simulink model "SatelliteServicing_3LinkPlanar - Copy"  (R2021a)
settings: Solver=ode15s  StartTime=0.0  StopTime=endTime  RelTol=1e-3
undefined symbols (not defined in the file or in its folder): alpha, Base_a, Base_c, Base_z, client, controlData, DiscIntNeverNeededParam, inertiaMat, inertiaMatBase, Link_Length, linkInertia, massVec, mt, nav, rod, sat, sigbuilder_block, smiData, X, Y, Z
libraries: nesl_utility x113, sm_lib x56
(part 3 of 3)

== system SatelliteServicing_3LinkPlanar - Copy/ServicingSatellite/SatSolarPanel2 ==
  Rigid Transform : sm_lib/Frames and Transforms/Rigid Transform  TranslationMethod=None  TranslationStandardOffset=0  TranslationLengthUnit=m  TranslationStandardAxis=+Z  TranslationCartesianOffset=[0 0 0]  TranslationROffset=0  TranslationROffsetUnits=m  TranslationZOffset=0  TranslationZOffsetUnits=m  TranslationThetaOffset=0  TranslationThetaOffsetUnits=deg  RotationMethod=RotationSequence  RotationAngleUnits=deg  RotationStandardAxis=+Z  RotationAngle=0.0  RotationArbitraryAxis=[0 0 1]  FollAlignAxisA=+X  BaseAlignAxisA=+Y  FollAlignAxisB=+Y  BaseAlignAxisB=+Z  RotationSequenceAxes=FollowerAxes  RotationSequence=YZX  RotationSequenceAngles=[0 90 0]  RotationSequenceAnglesUnits=deg  RotationMatrix=[1 0 0; 0 1 0; 0 0 1]
  SolarPanelSolid1 : sm_lib/Body Elements/Brick Solid  GraphicAmbientColor=[0.15 0.15 0.15 1.0]  BasedOnType=Mass  BrickDimensions=sat.service.panel_mount.dim  BrickDimensionUnits=m  CenterOfMass=[0 0 0]  CenterOfMassUnits=m  GraphicDiffuseColor=[0.2 0.2 0.2]  Density=1000  DensityUnits=kg/m^3  DoExposeReferenceFrame=off  GraphicEmissiveColor=[0.0 0.0 0.0 1.0]  ExportEntireGeometry=off  SerializedFrames=<Frames><Frame><Id>Frame1</Id><Value><Name>F1</Name><Origin><Source>GeometricFeature</Source><FeatureName>-x surface</FeatureName></Origin><PrimaryAxis><DefinedDirection>+Z</DefinedDirection><Source>ReferenceFrame</Source><SourceDirection>+Z</SourceDirection><FeatureName></FeatureName></PrimaryAxis><SecondaryAxis><DefinedDirection>+X</DefinedDirection><Source>ReferenceFrame</Source><SourceDirection>+X</SourceDirection><FeatureName></FeatureName></SecondaryAxis></Value></Frame><Frame><Id>Frame2</Id><Value><Name>F2</Name><Origin><Source>GeometricFeature</Source><FeatureName>+x surface</FeatureName></Origin><PrimaryAxis><DefinedDirection>+Z</DefinedDirection><Source>ReferenceFrame</Source><SourceDirection>+Z</SourceDirection><FeatureName></FeatureName></PrimaryAxis><SecondaryAxis><DefinedDirection>+X</DefinedDirection><Source>ReferenceFrame</Source><SourceDirection>+X</SourceDirection><FeatureName></FeatureName></SecondaryAxis></Value></Frame></Frames>  MarkerShape=Sphere  MarkerSize=10  GraphicType=FromGeometry  InertiaType=CalculateFromGeometry  Mass=sat.service.panel_mount.mass  MassUnits=kg  MomentsOfInertia=[1 1 1]  MomentsOfInertiaUnits=kg*m^2  GraphicOpacity=0.5  ProductsOfInertia=[0 0 0]  ProductsOfInertiaUnits=kg*m^2  GraphicShininess=75  GraphicSpecularColor=[0.5 0.5 0.5 1.0]  GraphicVisPropType=SimpleVisualProperties
  SolarPanelSolid2 : sm_lib/Body Elements/Brick Solid  GraphicAmbientColor=[0.15 0.15 0.15 1.0]  BasedOnType=Mass  BrickDimensions=sat.service.panel.dim  BrickDimensionUnits=m  CenterOfMass=[0 0 0]  CenterOfMassUnits=m  GraphicDiffuseColor=[0.0 0.2 0.8]  Density=1000  DensityUnits=kg/m^3  DoExposeReferenceFrame=off  GraphicEmissiveColor=[0.0 0.0 0.0 1.0]  ExportEntireGeometry=off  SerializedFrames=<Frames><Frame><Id>Frame1</Id><Value><Name>F1</Name><Origin><Source>GeometricFeature</Source><FeatureName>-x surface</FeatureName></Origin><PrimaryAxis><DefinedDirection>+Z</DefinedDirection><Source>ReferenceFrame</Source><SourceDirection>+Z</SourceDirection><FeatureName></FeatureName></PrimaryAxis><SecondaryAxis><DefinedDirection>+X</DefinedDirection><Source>ReferenceFrame</Source><SourceDirection>+X</SourceDirection><FeatureName></FeatureName></SecondaryAxis></Value></Frame></Frames>  MarkerShape=Sphere  MarkerSize=10  GraphicType=FromGeometry  InertiaType=CalculateFromGeometry  Mass=sat.service.panel.mass  MassUnits=kg  MomentsOfInertia=[1 1 1]  MomentsOfInertiaUnits=kg*m^2  GraphicOpacity=0.5  ProductsOfInertia=[0 0 0]  ProductsOfInertiaUnits=kg*m^2  GraphicShininess=75  GraphicSpecularColor=[0.5 0.5 0.5 1.0]  GraphicVisPropType=SimpleVisualProperties
  F1 : PMIOPort  Side=Left
  connections:
  SolarPanelSolid2/LConn1 -- SolarPanelSolid1/RConn1
  Rigid Transform/RConn1 -- SolarPanelSolid1/LConn1
  Rigid Transform/LConn1 -- F1/RConn1

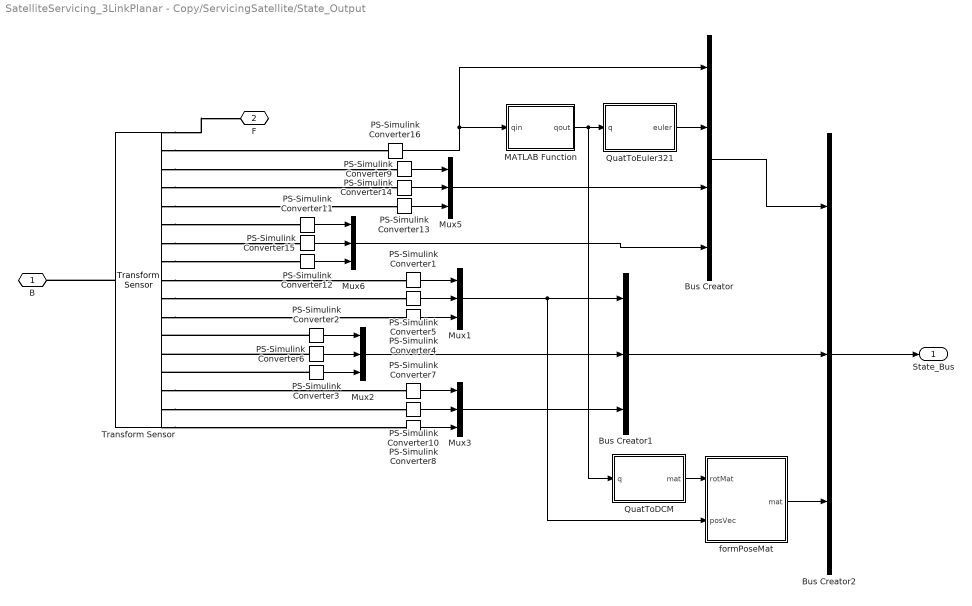
== system SatelliteServicing_3LinkPlanar - Copy/ServicingSatellite/State_Output ==
  Bus Creator : BusCreator  Inputs=4  OutDataTypeStr=Bus: RotStateBus
      settings: InheritFromInputs=off
  Bus Creator1 : BusCreator  Inputs=3  OutDataTypeStr=Bus: TransStateBus
      settings: InheritFromInputs=off
  Bus Creator2 : BusCreator  Inputs=3  OutDataTypeStr=Bus: StateBus
      settings: InheritFromInputs=off
  MATLAB Function : MATLAB Function  TreatAsAtomicUnit=on
  Mux{1..3,5..6} (5 alike) : Mux  Inputs=3
  PS-Simulink Converter{1..16} (16 alike) : nesl_utility/PS-Simulink Converter  PhysicalDomain=network_engine_domain  SubClassName=ps_output  LeftPortType=input  RightPortType=output  PseudoPeriodic=off  Frequencies=[]  Unit=inherit  AffineConversion=off
      settings: SourceProductBaseCode=PW,SS
  QuatToDCM : MATLAB Function  TreatAsAtomicUnit=on
  QuatToEuler321 : MATLAB Function  TreatAsAtomicUnit=on
  Transform Sensor : sm_lib/Frames and Transforms/Transform Sensor  MeasurementFrame=World  SenseAngle=off  SenseAxis=off  SenseAngle1=off  SenseAngle2=off  SenseAngle3=off  SenseQ=on  SenseR=off  SenseOmegaX=on  SenseOmegaY=on  SenseOmegaZ=on  SenseOmega1=off  SenseOmega2=off  SenseOmega3=off  SenseQDot=off  SenseRDot=off  SenseAlphaX=on  SenseAlphaY=on  SenseAlphaZ=on  SenseAlpha1=off  SenseAlpha2=off  SenseAlpha3=off  SenseQDDot=off  SenseRDDot=off  SenseX=on  SenseY=on  SenseZ=on  SenseRad=off  SenseAzim=off  SenseDist=off  SenseInc=off  SenseXDot=on  SenseYDot=on  SenseZDot=on  SenseRadDot=off  SenseAzimDot=off  SenseDistDot=off  SenseIncDot=off  SenseXDDot=on  SenseYDDot=on  SenseZDDot=on  SenseRadDDot=off  SenseAzimDDot=off  SenseDistDDot=off  SenseIncDDot=off
  formPoseMat : MATLAB Function  TreatAsAtomicUnit=on
  B : PMIOPort  Side=Left
  F : PMIOPort  Port=2  Side=Right
  State_Bus : Outport
  wires:
  PS-Simulink Converter4/1 -> Mux1/3
  PS-Simulink Converter5/1 -> Mux1/2
  PS-Simulink Converter1/1 -> Mux1/1
  PS-Simulink Converter3/1 -> Mux2/3
  PS-Simulink Converter6/1 -> Mux2/2
  PS-Simulink Converter2/1 -> Mux2/1
  PS-Simulink Converter10/1 -> Mux3/2
  PS-Simulink Converter8/1 -> Mux3/3
  PS-Simulink Converter7/1 -> Mux3/1
  Mux2/1 -> Bus Creator1/2
  Mux1/1 -> formPoseMat/2(posVec), Bus Creator1/1
  Mux3/1 -> Bus Creator1/3
  PS-Simulink Converter9/1 -> Mux5/1
  PS-Simulink Converter14/1 -> Mux5/2
  PS-Simulink Converter13/1 -> Mux5/3
  Mux5/1 -> Bus Creator/3
  PS-Simulink Converter15/1 -> Mux6/2
  PS-Simulink Converter12/1 -> Mux6/3
  Mux6/1 -> Bus Creator/4
  PS-Simulink Converter11/1 -> Mux6/1
  PS-Simulink Converter16/1 -> Bus Creator/1, MATLAB Function/1(qin)
  QuatToEuler321/1(euler) -> Bus Creator/2
  Bus Creator/1 -> Bus Creator2/1
  Bus Creator1/1 -> Bus Creator2/2
  Bus Creator2/1 -> State_Bus/1
  MATLAB Function/1(qout) -> QuatToDCM/1(q), QuatToEuler321/1(q)
  QuatToDCM/1(mat) -> formPoseMat/1(rotMat)
  formPoseMat/1(mat) -> Bus Creator2/3
  connections:
  Transform Sensor/LConn1 -- B/RConn1
  Transform Sensor/RConn1 -- F/RConn1
  Transform Sensor/RConn9 -- PS-Simulink Converter1/LConn1
  Transform Sensor/RConn10 -- PS-Simulink Converter5/LConn1
  Transform Sensor/RConn11 -- PS-Simulink Converter4/LConn1
  PS-Simulink Converter3/LConn1 -- Transform Sensor/RConn14
  PS-Simulink Converter6/LConn1 -- Transform Sensor/RConn13
  PS-Simulink Converter2/LConn1 -- Transform Sensor/RConn12
  Transform Sensor/RConn17 -- PS-Simulink Converter8/LConn1
  Transform Sensor/RConn15 -- PS-Simulink Converter7/LConn1
  Transform Sensor/RConn16 -- PS-Simulink Converter10/LConn1
  Transform Sensor/RConn8 -- PS-Simulink Converter12/LConn1
  Transform Sensor/RConn5 -- PS-Simulink Converter13/LConn1
  Transform Sensor/RConn4 -- PS-Simulink Converter14/LConn1
  Transform Sensor/RConn3 -- PS-Simulink Converter9/LConn1
  Transform Sensor/RConn7 -- PS-Simulink Converter15/LConn1
  Transform Sensor/RConn6 -- PS-Simulink Converter11/LConn1
  Transform Sensor/RConn2 -- PS-Simulink Converter16/LConn1

== system SatelliteServicing_3LinkPlanar - Copy/GNC/Control/MassProperties ==
  linkInertia : Inport
  Bus Creator : BusCreator  Inputs=5  OutDataTypeStr=Bus: MassPropertiesBus
      settings: InheritFromInputs=off
  Constant10 : Constant  Value=massVec
  Constant11 : Constant  Value=mt
  Constant12 : Constant  Value=inertiaMatBase
  Constant13 : Constant  Value=inertiaMat
  InitialMP : Outport
  wires:
  Constant11/1 -> Bus Creator/1
  Constant10/1 -> Bus Creator/2
  Constant12/1 -> Bus Creator/3
  Constant13/1 -> Bus Creator/4
  Bus Creator/1 -> InitialMP/1
  ? -> Bus Creator/5

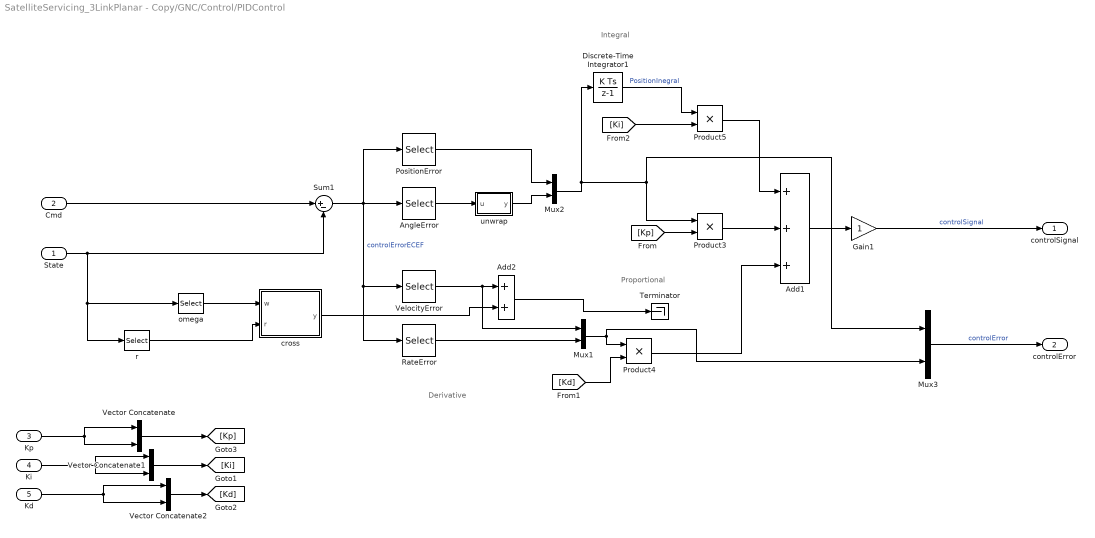
== system SatelliteServicing_3LinkPlanar - Copy/GNC/Control/PIDControl ==
  note: Derivative
  note: Proportional
  note: Integral
  State : Inport
  Cmd : Inport  Port=2
  Kp : Inport  Port=3
  Ki : Inport  Port=4
  Kd : Inport  Port=5
  Add1 : Sum  Inputs=+++
  Add2 : Sum
  AngleError : Selector  IndexOptions=Index vector (dialog)  Indices=[4:6]  OutputSizes=1
  Discrete-Time Integrator1 : DiscreteIntegrator  SampleTime=-1  ICPrevOutput=DiscIntNeverNeededParam  ICPrevScaledInput=DiscIntNeverNeededParam
  Gain1 : Gain
  Mux1 : Mux  Inputs=2
  Mux2 : Mux  Inputs=2
  Mux3 : Mux  Inputs=2
  PositionError : Selector  IndexOptions=Index vector (dialog)  Indices=[1:3]  OutputSizes=1
  Product3 : Product
  Product4 : Product
  Product5 : Product
  RateError : Selector  IndexOptions=Index vector (dialog)  Indices=[10:12]  OutputSizes=1
  Sum1 : Sum  Inputs=|+-
  Terminator : Terminator
  Vector Concatenate : Concatenate
  Vector Concatenate1 : Concatenate
  Vector Concatenate2 : Concatenate
  VelocityError : Selector  IndexOptions=Index vector (dialog)  Indices=[7:9]  OutputSizes=1
  cross : MATLAB Function  TreatAsAtomicUnit=on
  omega : Selector  IndexOptions=Index vector (dialog)  Indices=[10:12]  OutputSizes=1
  r : Selector  IndexOptions=Index vector (dialog)  Indices=[1:3]  OutputSizes=1
  unwrap : MATLAB Function  TreatAsAtomicUnit=on
  controlSignal : Outport
  controlError : Outport  Port=2
  wires:
  Mux2/1 -> Discrete-Time Integrator1/1, Product3/1, Mux3/1
  Product3/1 -> Add1/2
  Sum1/1 -> VelocityError/1, RateError/1, AngleError/1, PositionError/1  "controlErrorECEF"
  Discrete-Time Integrator1/1 -> Product5/1  "PositionInegral"
  RateError/1 -> Mux1/2
  Product5/1 -> Add1/1
  State/1 -> r/1, omega/1, Sum1/2
  Gain1/1 -> controlSignal/1  "controlSignal"
  cross/1(y) -> Add2/2
  PositionError/1 -> Mux2/1
  Mux1/1 -> Product4/1, Mux3/2
  Mux3/1 -> controlError/1  "controlError"
  [Ki] -> Product5/2
  r/1 -> cross/2(r)
  [Kp] -> Product3/2
  [Kd] -> Product4/2
  AngleError/1 -> unwrap/1(u)
  omega/1 -> cross/1(w)
  Add1/1 -> Gain1/1
  Product4/1 -> Add1/3
  Cmd/1 -> Sum1/1
  VelocityError/1 -> Mux1/1, Add2/1
  Kp/1 -> Vector Concatenate/1, Vector Concatenate/2
  Vector Concatenate/1 -> [Kp]
  Vector Concatenate2/1 -> [Kd]
  Kd/1 -> Vector Concatenate2/2, Vector Concatenate2/1
  Vector Concatenate1/1 -> [Ki]
  Ki/1 -> Vector Concatenate1/2, Vector Concatenate1/1
  Add2/1 -> Terminator/1
  unwrap/1(y) -> Mux2/2

== system SatelliteServicing_3LinkPlanar - Copy/GNC/Motion Inputs/SatMotion_fz ==
  Demux : Demux  Tag=STV Demux  Outputs=1
      settings: DisplayOption=none
  FromWs : FromWorkspace  Tag=STV FromWs  VariableName=tuvar
      SigBuilderData=|
      | common.afterFinalStr = 'Extrapolate'
      | common.sampleTime = 0
      | dataSet.timeRange = [0 13]
      | dataSet.name = 'Group 1'
      | sbobj.Groups.Name = 'Group 1'
      | sbobj.Groups.Signals.Name = 'SatMotion_fz'
      | sbobj.Groups.Signals.XData = [0 1 1 1.5 1.5 13]
      | sbobj.Groups.Signals.YData = [0 0 20 20 0 0]
      | sbobj.Groups.TimeRange = [0 13]
  SatMotion_fz : Outport  Tag=STV Outport
  wires:
  FromWs/1 -> Demux/1
  Demux/1 -> SatMotion_fz/1

== system SatelliteServicing_3LinkPlanar - Copy/GNC/Navigation/ComputeRelativePose ==
  Rel_to_Camera : Inport
  Bus Selector2 : BusSelector  OutputSignals=poseMatrix
  Constant1 : Constant  Value=nav.CameraToBase.orientation
  Constant2 : Constant  Value=[0 0 0]
  Product : Product  Multiplication=Matrix(*)
  Reshape : Reshape  OutputDimensionality=Column vector (2-D)
  Selector : Selector  NumberOfDimensions=2  InputPortWidth=3  IndexOptions=Index vector (dialog),Index vector (dialog)  Indices=[1:3],[1:3]  OutputSizes=1,1
  To Workspace1 : ToWorkspace  VariableName=euler_cameraAttach  SaveFormat=Timeseries  SampleTime=-1
  To Workspace2 : ToWorkspace  VariableName=mat_cameraBody  SaveFormat=Timeseries  SampleTime=-1
  formPoseMat : MATLAB Function  TreatAsAtomicUnit=on
  formRotMat : MATLAB Function  TreatAsAtomicUnit=on
  formRotMat1 : MATLAB Function  TreatAsAtomicUnit=on
  "Rel_to_CameraAttach " : Outport
  wires:
  formRotMat/1(mat) -> To Workspace2/1, formPoseMat/1(rotMat)
  Rel_to_Camera/1 -> Bus Selector2/1
  Product/1 -> Selector/1, "Rel_to_CameraAttach "/1
  Selector/1 -> formRotMat1/1(mat)
  formRotMat1/1(euler) -> To Workspace1/1
  Constant2/1 -> Reshape/1
  Reshape/1 -> formPoseMat/2(posVec)
  Constant1/1 -> formRotMat/1(euler)
  formPoseMat/1(mat) -> Product/2
  Bus Selector2/1 -> Product/1  "<poseMatrix>"

== system SatelliteServicing_3LinkPlanar - Copy/RoboticArm/ArmSegmentAssembly_2/ArmSegment_1_RIGID ==
  ReferenceFrame : sm_lib/Frames and Transforms/Reference Frame
  Solid : sm_lib/Body Elements/File Solid  ExtGeomFileName=ArmSegment_Default_sldprt.STEP  UnitType=FromFile  ExtGeomFileUnits=m  StepReaderType=HEX  ExportConvexHullGeometry=off  InertiaType=Custom  Mass=smiData.Solid(2).mass  MassUnits=kg  CenterOfMass=smiData.Solid(2).CoM  CenterOfMassUnits=mm  MomentsOfInertia=smiData.Solid(2).MoI  MomentsOfInertiaUnits=kg*mm^2  ProductsOfInertia=smiData.Solid(2).PoI  ProductsOfInertiaUnits=kg*mm^2  BasedOnType=DensityFromFile  Density=1000  DensityUnits=kg/m^3  DoExposeReferenceFrame=off  SerializedFrames=<Frames><Frame><Id>Frame1</Id><Value><Name>J1</Name><Origin><Source>GeometricFeature</Source><FeatureName>segment 68</FeatureName></Origin><PrimaryAxis><DefinedDirection>+Z</DefinedDirection><Source>ReferenceFrame</Source><SourceDirection>+Y</SourceDirection><FeatureName></FeatureName></PrimaryAxis><SecondaryAxis><DefinedDirection>+X</DefinedDirection><Source>ReferenceFrame</Source><SourceDirection>+X</SourceDirection><FeatureName></FeatureName></SecondaryAxis></Value></Frame><Frame><Id>Frame2</Id><Value><Name>J2</Name><Origin><Source>GeometricFeature</Source><FeatureName>circular curve 16</FeatureName></Origin><PrimaryAxis><DefinedDirection>+Z</DefinedDirection><Source>ReferenceFrame</Source><SourceDirection>+Y</SourceDirection><FeatureName></FeatureName></PrimaryAxis><SecondaryAxis><DefinedDirection>+X</DefinedDirection><Source>ReferenceFrame</Source><SourceDirection>+X</SourceDirection><FeatureName></FeatureName></SecondaryAxis></Value></Frame></Frames>  GraphicType=FromGeometry  MarkerShape=Sphere  MarkerSize=10  GraphicVisPropType=SimpleVisualProperties  GraphicDiffuseColor=smiData.Solid(2).color  GraphicSpecularColor=[0.5 0.5 0.5 1.0]  GraphicAmbientColor=[0.15 0.15 0.15 1.0]  GraphicEmissiveColor=[0.0 0.0 0.0 1.0]  GraphicShininess=75  GraphicOpacity=smiData.Solid(2).opacity
  Transform : sm_lib/Frames and Transforms/Rigid Transform  TranslationMethod=Cartesian  TranslationStandardOffset=0  TranslationLengthUnit=mm  TranslationStandardAxis=+Z  TranslationCartesianOffset=smiData.RigidTransform(5).translation  TranslationROffset=0  TranslationROffsetUnits=m  TranslationZOffset=0  TranslationZOffsetUnits=m  TranslationThetaOffset=0  TranslationThetaOffsetUnits=deg  RotationMethod=ArbitraryAxis  RotationAngleUnits=rad  RotationStandardAxis=+Z  RotationAngle=smiData.RigidTransform(5).angle  RotationArbitraryAxis=smiData.RigidTransform(5).axis  FollAlignAxisA=+X  BaseAlignAxisA=+Y  FollAlignAxisB=+Y  BaseAlignAxisB=+Z  RotationSequenceAxes=FollowerAxes  RotationSequence=XYX  RotationSequenceAngles=[0 0 0]  RotationSequenceAnglesUnits=deg  RotationMatrix=[1 0 0; 0 1 0; 0 0 1]
  Transform1 : sm_lib/Frames and Transforms/Rigid Transform  TranslationMethod=Cartesian  TranslationStandardOffset=0  TranslationLengthUnit=mm  TranslationStandardAxis=+Z  TranslationCartesianOffset=smiData.RigidTransform(4).translation  TranslationROffset=0  TranslationROffsetUnits=m  TranslationZOffset=0  TranslationZOffsetUnits=m  TranslationThetaOffset=0  TranslationThetaOffsetUnits=deg  RotationMethod=ArbitraryAxis  RotationAngleUnits=rad  RotationStandardAxis=+Z  RotationAngle=smiData.RigidTransform(4).angle  RotationArbitraryAxis=smiData.RigidTransform(4).axis  FollAlignAxisA=+X  BaseAlignAxisA=+Y  FollAlignAxisB=+Y  BaseAlignAxisB=+Z  RotationSequenceAxes=FollowerAxes  RotationSequence=XYX  RotationSequenceAngles=[0 0 0]  RotationSequenceAnglesUnits=deg  RotationMatrix=[1 0 0; 0 1 0; 0 0 1]
  J1_2 : PMIOPort  Side=Left
  J2_1 : PMIOPort  Port=2  Side=Right
  connections:
  Transform/RConn1 -- J2_1/RConn1
  Transform/LConn1 -- Solid/RConn1
  J1_2/RConn1 -- Transform1/LConn1
  Solid/LConn1 -- ReferenceFrame/RConn1 -- Transform1/RConn1

== system SatelliteServicing_3LinkPlanar - Copy/RoboticArm/ArmSegmentAssembly_3/ArmSegment_1_RIGID ==
  ReferenceFrame : sm_lib/Frames and Transforms/Reference Frame
  Solid : sm_lib/Body Elements/File Solid  ExtGeomFileName=ArmSegment_Default_sldprt.STEP  UnitType=FromFile  ExtGeomFileUnits=m  StepReaderType=HEX  ExportConvexHullGeometry=off  InertiaType=Custom  Mass=smiData.Solid(3).mass  MassUnits=kg  CenterOfMass=smiData.Solid(3).CoM  CenterOfMassUnits=mm  MomentsOfInertia=smiData.Solid(3).MoI  MomentsOfInertiaUnits=kg*mm^2  ProductsOfInertia=smiData.Solid(3).PoI  ProductsOfInertiaUnits=kg*mm^2  BasedOnType=DensityFromFile  Density=1000  DensityUnits=kg/m^3  DoExposeReferenceFrame=off  SerializedFrames=<Frames><Frame><Id>Frame1</Id><Value><Name>J2</Name><Origin><Source>GeometricFeature</Source><FeatureName>segment 68</FeatureName></Origin><PrimaryAxis><DefinedDirection>+Z</DefinedDirection><Source>ReferenceFrame</Source><SourceDirection>+Y</SourceDirection><FeatureName></FeatureName></PrimaryAxis><SecondaryAxis><DefinedDirection>+X</DefinedDirection><Source>ReferenceFrame</Source><SourceDirection>+X</SourceDirection><FeatureName></FeatureName></SecondaryAxis></Value></Frame><Frame><Id>Frame2</Id><Value><Name>J3</Name><Origin><Source>GeometricFeature</Source><FeatureName>circular curve 13</FeatureName></Origin><PrimaryAxis><DefinedDirection>+Z</DefinedDirection><Source>ReferenceFrame</Source><SourceDirection>+Y</SourceDirection><FeatureName></FeatureName></PrimaryAxis><SecondaryAxis><DefinedDirection>+X</DefinedDirection><Source>ReferenceFrame</Source><SourceDirection>+X</SourceDirection><FeatureName></FeatureName></SecondaryAxis></Value></Frame></Frames>  GraphicType=FromGeometry  MarkerShape=Sphere  MarkerSize=10  GraphicVisPropType=SimpleVisualProperties  GraphicDiffuseColor=smiData.Solid(2).color  GraphicSpecularColor=[0.5 0.5 0.5 1.0]  GraphicAmbientColor=[0.15 0.15 0.15 1.0]  GraphicEmissiveColor=[0.0 0.0 0.0 1.0]  GraphicShininess=75  GraphicOpacity=smiData.Solid(2).opacity
  Transform : sm_lib/Frames and Transforms/Rigid Transform  TranslationMethod=Cartesian  TranslationStandardOffset=0  TranslationLengthUnit=mm  TranslationStandardAxis=+Z  TranslationCartesianOffset=smiData.RigidTransform(6).translation  TranslationROffset=0  TranslationROffsetUnits=m  TranslationZOffset=0  TranslationZOffsetUnits=m  TranslationThetaOffset=0  TranslationThetaOffsetUnits=deg  RotationMethod=ArbitraryAxis  RotationAngleUnits=rad  RotationStandardAxis=+Z  RotationAngle=smiData.RigidTransform(6).angle  RotationArbitraryAxis=smiData.RigidTransform(6).axis  FollAlignAxisA=+X  BaseAlignAxisA=+Y  FollAlignAxisB=+Y  BaseAlignAxisB=+Z  RotationSequenceAxes=FollowerAxes  RotationSequence=XYX  RotationSequenceAngles=[0 0 0]  RotationSequenceAnglesUnits=deg  RotationMatrix=[1 0 0; 0 1 0; 0 0 1]
  Transform1 : sm_lib/Frames and Transforms/Rigid Transform  TranslationMethod=Cartesian  TranslationStandardOffset=0  TranslationLengthUnit=mm  TranslationStandardAxis=+Z  TranslationCartesianOffset=smiData.RigidTransform(7).translation  TranslationROffset=0  TranslationROffsetUnits=m  TranslationZOffset=0  TranslationZOffsetUnits=m  TranslationThetaOffset=0  TranslationThetaOffsetUnits=deg  RotationMethod=ArbitraryAxis  RotationAngleUnits=rad  RotationStandardAxis=+Z  RotationAngle=smiData.RigidTransform(7).angle  RotationArbitraryAxis=smiData.RigidTransform(7).axis  FollAlignAxisA=+X  BaseAlignAxisA=+Y  FollAlignAxisB=+Y  BaseAlignAxisB=+Z  RotationSequenceAxes=FollowerAxes  RotationSequence=XYX  RotationSequenceAngles=[0 0 0]  RotationSequenceAnglesUnits=deg  RotationMatrix=[1 0 0; 0 1 0; 0 0 1]
  J2_2 : PMIOPort  Side=Left
  J3_1 : PMIOPort  Port=2  Side=Right
  connections:
  Transform1/RConn1 -- J3_1/RConn1
  ReferenceFrame/RConn1 -- Solid/RConn1 -- Transform1/LConn1
  J2_2/RConn1 -- Transform/LConn1
  Transform/RConn1 -- Solid/LConn1

== matlab function SatelliteServicing_3LinkPlanar - Copy/ServicingSatellite/State_Output/QuatToEuler321 ==
  data: q input; euler output
function euler  = callQuatToEuler321(q)


[euler] = quatToEuler_321(q);

== matlab function SatelliteServicing_3LinkPlanar - Copy/GNC/Control/PIDControl/cross ==
  data: y output; w input; r input
function y  = fcn(w,r)


y = cross(w,r);

== matlab function SatelliteServicing_3LinkPlanar - Copy/ServicingSatellite/State_Output/MATLAB Function ==
  data: qin input; qout output
function qout = call_quatconj(qin)

qout = zeros(1,4);
qout = quatconj(qin');

== matlab function SatelliteServicing_3LinkPlanar - Copy/ServicingSatellite/State_Output/QuatToDCM ==
  data: q input; mat output
function mat  = callQuatToDCM(q)

[mat] = quatToDCM(q);

== matlab function SatelliteServicing_3LinkPlanar - Copy/ServicingSatellite/State_Output/formPoseMat ==
  data: rotMat input; mat output; posVec input
function mat  = callFormPoseMat(rotMat,posVec)


[mat] = formPoseMat(rotMat,posVec);

== matlab function SatelliteServicing_3LinkPlanar - Copy/RoboticArm/State_Output2/QuatToEuler321 ==
  data: q input; euler output
function euler  = callQuatToEuler321(q)


[euler] = quatToEuler_321(q);

== matlab function SatelliteServicing_3LinkPlanar - Copy/RoboticArm/State_Output2/formPoseMat ==
  data: rotMat input; mat output; posVec input
function mat  = callFormPoseMat(rotMat,posVec)


[mat] = formPoseMat(rotMat,posVec);

== matlab function SatelliteServicing_3LinkPlanar - Copy/RoboticArm/State_Output1/MATLAB Function ==
  data: qin input; qout output
function qout = call_quatconj(qin)

qout = zeros(1,4);
qout = quatconj(qin');

== matlab function SatelliteServicing_3LinkPlanar - Copy/RoboticArm/State_Output1/QuatToDCM ==
  data: q input; mat output
function mat  = callQuatToDCM(q)

[mat] = quatToDCM(q);

== matlab function SatelliteServicing_3LinkPlanar - Copy/RoboticArm/State_Output1/QuatToEuler321 ==
  data: q input; euler output
function euler  = callQuatToEuler321(q)


[euler] = quatToEuler_321(q);

== matlab function SatelliteServicing_3LinkPlanar - Copy/RoboticArm/State_Output1/formPoseMat ==
  data: rotMat input; mat output; posVec input
function mat  = callFormPoseMat(rotMat,posVec)


[mat] = formPoseMat(rotMat,posVec);

== matlab function SatelliteServicing_3LinkPlanar - Copy/ClientSatellite/State_Output2/MATLAB Function ==
  data: qin input; qout output
function qout = call_quatconj(qin)

qout = zeros(1,4);
qout = quatconj(qin');

== matlab function SatelliteServicing_3LinkPlanar - Copy/RelativeState/State_Output2/QuatToDCM ==
  data: q input; mat output
function mat  = callQuatToDCM(q)

[mat] = simscapeQuatToDCM(q);

== matlab function SatelliteServicing_3LinkPlanar - Copy/RelativeState/State_Output2/QuatToEuler321 ==
  data: q input; euler output
function euler  = callQuatToEuler321(q)


[euler] = quatToEuler_321(q);

== matlab function SatelliteServicing_3LinkPlanar - Copy/RelativeState/State_Output2/formPoseMat ==
  data: rotMat input; mat output; posVec input
function mat  = callFormPoseMat(rotMat,posVec)


[mat] = formPoseMat(rotMat,posVec);

== matlab function SatelliteServicing_3LinkPlanar - Copy/GNC/Navigation/ComputeRelativePose/formRotMat1 ==
  data: mat input; euler output
function euler  = callDCMToEuler(mat)

[euler] = DCMToEuler_321(mat);

== matlab function SatelliteServicing_3LinkPlanar - Copy/ClientSatellite/State_Output2/QuatToDCM ==
  data: q input; mat output
function mat  = callQuatToDCM(q)

[mat] = quatToDCM(q);

== matlab function SatelliteServicing_3LinkPlanar - Copy/ClientSatellite/State_Output2/QuatToEuler321 ==
  data: q input; euler output
function euler  = callQuatToEuler321(q)


[euler] = quatToEuler_321(q);

== matlab function SatelliteServicing_3LinkPlanar - Copy/ClientSatellite/State_Output2/formPoseMat ==
  data: rotMat input; mat output; posVec input
function mat  = callFormPoseMat(rotMat,posVec)


[mat] = formPoseMat(rotMat,posVec);

== matlab function SatelliteServicing_3LinkPlanar - Copy/ClientSatellite/State_Output/MATLAB Function ==
  data: qin input; qout output
function qout = call_quatconj(qin)

qout = zeros(1,4);
qout = quatconj(qin');

== matlab function SatelliteServicing_3LinkPlanar - Copy/ClientSatellite/State_Output/QuatToDCM ==
  data: q input; mat output
function mat  = callQuatToDCM(q)

[mat] = quatToDCM(q);

== matlab function SatelliteServicing_3LinkPlanar - Copy/ClientSatellite/State_Output/QuatToEuler321 ==
  data: q input; euler output
function euler  = callQuatToEuler321(q)


[euler] = quatToEuler_321(q);

== matlab function SatelliteServicing_3LinkPlanar - Copy/ClientSatellite/State_Output/formPoseMat ==
  data: rotMat input; mat output; posVec input
function mat  = callFormPoseMat(rotMat,posVec)


[mat] = formPoseMat(rotMat,posVec);

== matlab function SatelliteServicing_3LinkPlanar - Copy/RoboticArm/State_Output2/MATLAB Function ==
  data: qin input; qout output
function qout = call_quatconj(qin)

qout = zeros(1,4);
qout = quatconj(qin');

== matlab function SatelliteServicing_3LinkPlanar - Copy/RoboticArm/State_Output2/QuatToDCM ==
  data: q input; mat output
function mat  = callQuatToDCM(q)

[mat] = quatToDCM(q);

== matlab function SatelliteServicing_3LinkPlanar - Copy/GNC/Control/ArmKinematics ==
  data: Hstar output; Jstar output; cstar output; x0 input; geometry input Bus: GeometryBus; Link_Length input; massProperties input Bus: MassPropertiesBus; NLINKS parameter; linkInertia output
function [Hstar,Jstar,cstar,linkInertia] = call_armKinematics(x0,geometry,Link_Length,massProperties,NLINKS)


                                
[linkInertia,momentum,Hstar,Jstar,cstar] = armKinematics(x0,geometry,NLINKS,Link_Length,massProperties);

== matlab function SatelliteServicing_3LinkPlanar - Copy/GNC/Control/ComputeGeometry ==
  data: geometry output Bus: GeometryBus; x0 input; Link_Length input; massVec input; alpha input; Base_a input; Base_c input; Base_z input; NLINKS parameter
function geometry = call_computeGeometry(x0,Link_Length,massVec,alpha,Base_a,Base_c,Base_z, NLINKS)

%[geometryX,rVec,pVec,rVec0,rBase,RL,RLbase,RJ,RJbase,kVec,T00,PoseMats,alphaOut] = computeGeometry(x0,nLink,Link_Length,massVec,alpha,Base_a,Base_c,Base_z);
[geometry] = computeGeometry(x0,NLINKS,Link_Length,massVec,alpha,Base_a,Base_c,Base_z);

== matlab function SatelliteServicing_3LinkPlanar - Copy/GNC/Navigation/ComputeRelativePose/formPoseMat ==
  data: rotMat input; mat output; posVec input
function mat  = callFormPoseMat(rotMat,posVec)


[mat] = formPoseMat(rotMat,posVec);

== matlab function SatelliteServicing_3LinkPlanar - Copy/GNC/Navigation/ComputeRelativePose/formRotMat ==
  data: euler input; mat output
function mat  = callEulerToDCM(euler)

[mat] = EulerToDCM_321(euler);

== matlab function SatelliteServicing_3LinkPlanar - Copy/GNC/Control/computeTorque ==
  data: Hstar input; tau output; Jstar input; cstar input; controlSignal input
function tau  = computeTorque(Hstar,Jstar,cstar,controlSignal)

%tau = zeros(NLINKS,1);

JstarInv = pinv(Jstar);
qAngles = JstarInv*controlSignal';

tau = Hstar*qAngles + cstar';

== matlab function SatelliteServicing_3LinkPlanar - Copy/GNC/Control/PIDControl/unwrap ==
  data: y output; u input
function y  = fcn(u)


y = unwrap(u);
